simulink model "control_lab_2"  (R2016b)
settings: Solver=VariableStepAuto  StartTime=0.0  StopTime=10.0  RelTol=1e-3  EnableMultiTasking=on
values from neighbouring files (symbols this model uses):
  K = gain(x)    [radar_sweep.m]    (also in sweep.m; sweep_1.m; sweep_2.m; wind_sweep.m)
settings Model: Creator=zceehaq  LastModifiedBy=ammar_laptop
settings OptimizationCC: LifeSpan=inf
settings DebuggingCC: SFUnexpectedBacktrackingDiag=warning  SFNoUnconditionalDefaultTransitionDiag=warning  SFExecutionAtInitializationDiag=none
settings GRTTargetCC: TargetLangStandard=C89/C90 (ANSI)  GeneratePreprocessorConditionals=Disable all
settings ConfigComp: CovMetricSettings=dw  CovHtmlReporting=on  CovSaveCumulativeToWorkspaceVar=on  CovSaveSingleToWorkspaceVar=on  CovExternalEMLEnable=off

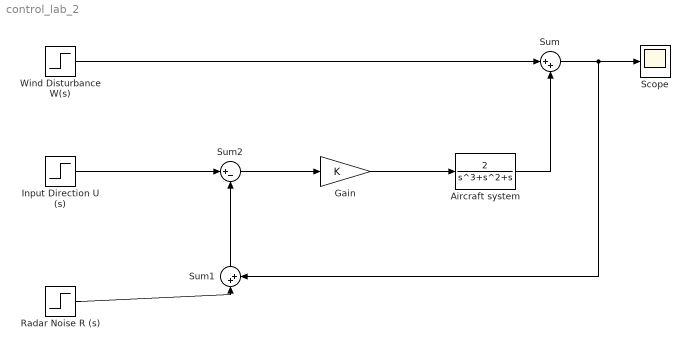
== system control_lab_2 ==
  "Aircraft system " : TransferFcn  Numerator=[2]  Denominator=[1 1 1 0]
  Gain : Gain  Gain=K
  Input Direction U (s) : Step  After=100  SampleTime=0
  Radar Noise R (s) : Step  SampleTime=0
  Scope : Scope
  Sum : Sum  Inputs=|++
  Sum1 : Sum  Inputs=|++
  Sum2 : Sum  Inputs=|+-
  Wind Disturbance W(s) : Step  SampleTime=0
  wires:
  Wind Disturbance W(s)/1 -> Sum/1
  Gain/1 -> "Aircraft system "/1
  "Aircraft system "/1 -> Sum/2
  Input Direction U (s)/1 -> Sum2/1
  Sum2/1 -> Gain/1
  Sum1/1 -> Sum2/2
  Sum/1 -> Sum1/2, Scope/1
  Radar Noise R (s)/1 -> Sum1/1
